simulink model "directional_control"  (R2020a)
settings: Solver=VariableStepAuto  StartTime=0.0  StopTime=50  RelTol=1e-3
undefined symbols (not defined in the file): den, num_zeta
settings Model: Creator=lum  LastModifiedBy=lum

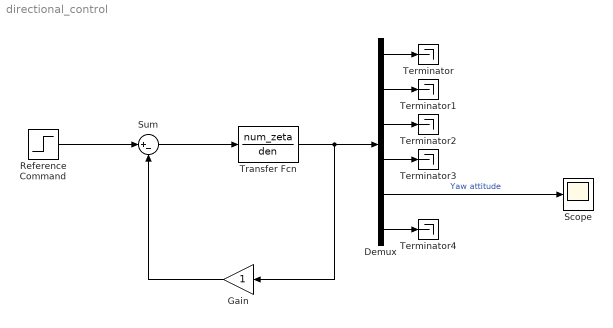
== system directional_control ==
  Demux : Demux  Outputs=6
  Gain : Gain
  Reference Command : Step  Time=0  After=deg2rad(1)  SampleTime=0
  Scope : Scope
  Sum : Sum  Inputs=|+-
  Terminator{,1..4} (5 alike) : Terminator
  Transfer Fcn : TransferFcn  Numerator=num_zeta  Denominator=den
  wires:
  Transfer Fcn/1 -> Gain/1, Demux/1
  Demux/1 -> Terminator/1
  Demux/2 -> Terminator1/1
  Demux/3 -> Terminator2/1
  Demux/4 -> Terminator3/1
  Demux/6 -> Terminator4/1
  Demux/5 -> Scope/1  "Yaw attitude"
  Sum/1 -> Transfer Fcn/1
  Reference Command/1 -> Sum/1
  Gain/1 -> Sum/2
